simulink model "ToLinearize"  (R2018a)
settings: Solver=VariableStepAuto  StartTime=0.0  StopTime=100  RelTol=1e-3
values from neighbouring files (symbols this model uses):
  B_p = 0.01325    [heli_parameters.m]
  B_y = 0.8513    [heli_parameters.m]
  F_cpp = 1    [heli_parameters.m]
  F_cpy = 1    [heli_parameters.m]
  F_cyp = 1    [heli_parameters.m]
  F_cyy = 1    [heli_parameters.m]
  g = 9.81    [Spoustec_simu.m]    (also in heli_parameters.m)
  h = 0.00714    [Spoustec_simu.m]    (also in heli_parameters.m)
  J_eqp = 0.0332    [heli_parameters.m]
  J_eqy = 0.0371    [heli_parameters.m]
  K_pp = 0.02638    [heli_parameters.m]
  K_py = 0.00189    [heli_parameters.m]
  K_yp = 0.002096    [heli_parameters.m]
  K_yy = 0.01871    [heli_parameters.m]
  l_mc = 0.0122    [heli_parameters.m]
  m = 1.3872    [Spoustec_simu.m]    (also in heli_parameters.m)
libraries: mpclib x2, cstblocks x1
settings Model: Creator=ja  LastModifiedBy=ja

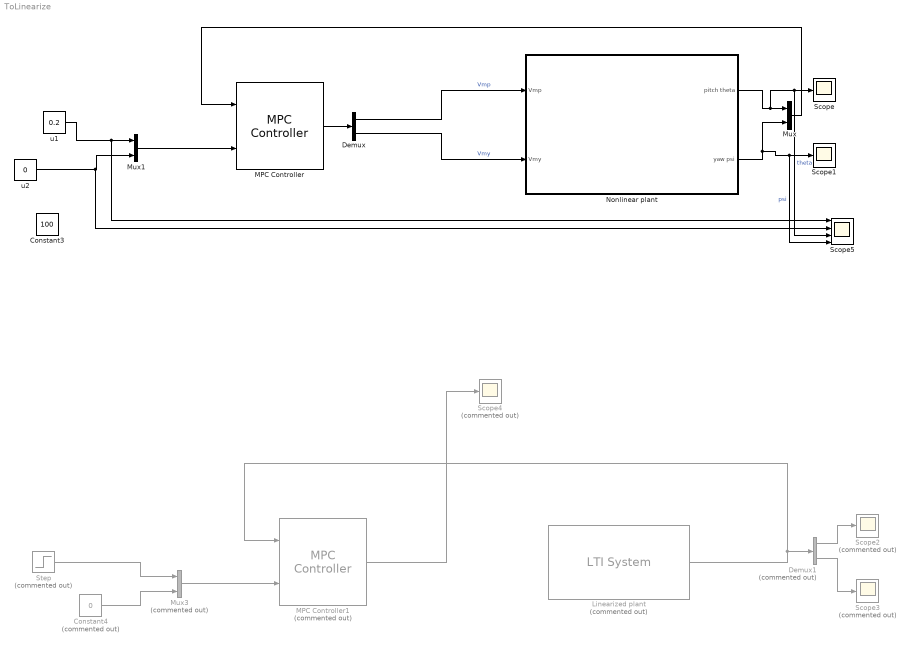
== system ToLinearize ==
  Constant3 : Constant  Value=100
  Constant4 : Constant  Commented=on  Value=0
  Demux : Demux  Outputs=2
  Demux1 : Demux  Commented=on  Outputs=2
  Linearized plant : cstblocks/LTI System  Commented=on  sys=plant  IC=[]
  MPC Controller : mpclib/MPC Controller  SCDEnableBlockLinearizationSpecification=on  mpcobj=mpc1  is_multiple=0  enable_value=0  return_u0=off  updateMPCinCallerWorkspace=on  ref_from_ws=off  ref_signal_name=[]  ref_preview=off  md_from_ws=off  md_signal_name=[]  md_preview=off  from_project=off  project_file=MPCtask.mat  md_inport=off  mv_inport=off  cost_outport=off  return_sequence=off  return_qpstatus=off  return_state=off  state_inport=off  lims_inport=off  cc_inport=off  ywt_inport=off  is_designfromscratch=0  uwt_inport=off  duwt_inport=off  rhoeps_inport=off  uref_inport=off  n_ts=1  n_p=20  n_mv=2  n_md=0  n_ud=0  n_mo=2  n_uo=0  BlockDataType=double  SampleTimeInherited=off  switch_inport=off
  MPC Controller1 : mpclib/MPC Controller  Commented=on  SCDEnableBlockLinearizationSpecification=on  is_multiple=0  enable_value=0  return_u0=off  updateMPCinCallerWorkspace=on  ref_from_ws=off  ref_signal_name=[]  ref_preview=off  md_from_ws=off  md_signal_name=[]  md_preview=off  from_project=off  project_file=MPCtask.mat  md_inport=off  mv_inport=off  cost_outport=off  return_sequence=off  return_qpstatus=off  return_state=off  state_inport=off  lims_inport=off  cc_inport=off  ywt_inport=off  is_designfromscratch=0  uwt_inport=off  duwt_inport=off  rhoeps_inport=off  uref_inport=off  n_ts=1  n_p=20  n_mv=2  n_md=0  n_ud=0  n_mo=2  n_uo=0  BlockDataType=double  SampleTimeInherited=off  switch_inport=off
  Mux : Mux  Inputs=2
  Mux1 : Mux  Inputs=2
  Mux3 : Mux  Commented=on  Inputs=2
  Nonlinear plant : Subsystem
      mask Display: image('Dynamics-of-2DOF-Helicopter.png');
  Scope : Scope
  Scope1 : Scope
  Scope2 : Scope  Commented=on
  Scope3 : Scope  Commented=on
  Scope4 : Scope  Commented=on
  Scope5 : Scope  NumInputPorts=4
  Step : Step  Commented=on  After=0.5  SampleTime=0
  u1 : Constant  Value=0.2
  u2 : Constant  Value=0
  wires:
  Demux/1 -> Nonlinear plant/1("Vmp ")  "Vmp"
  Demux/2 -> Nonlinear plant/2("Vmy ")  "Vmy"
  Nonlinear plant/1(pitch theta) -> Scope5/3, Scope/1, Mux/1  "theta"
  Nonlinear plant/2("yaw psi ") -> Scope5/4, Scope1/1, Mux/2  "psi"
  Mux/1 -> MPC Controller/1
  Mux1/1 -> MPC Controller/2
  u2/1 -> Scope5/2, Mux1/2
  Mux3/1 -> MPC Controller1/2
  Linearized plant/1 -> Demux1/1, MPC Controller1/1
  Step/1 -> Mux3/1
  Constant4/1 -> Mux3/2
  Demux1/1 -> Scope2/1
  Demux1/2 -> Scope3/1
  MPC Controller1/1 -> Scope4/1
  MPC Controller/1 -> Demux/1
  u1/1 -> Scope5/1, Mux1/1

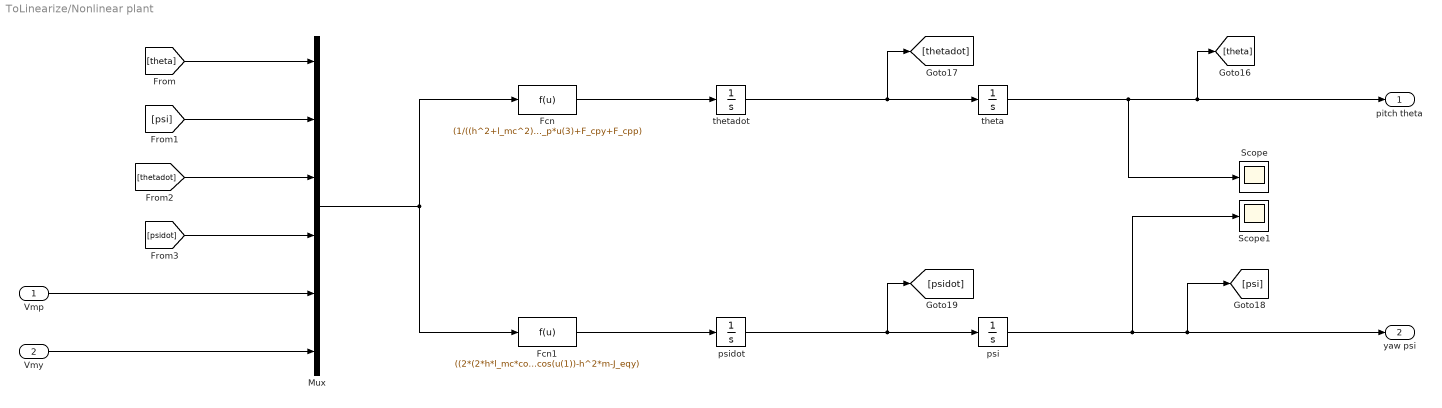
== system ToLinearize/Nonlinear plant ==
  "Vmp " : Inport
  "Vmy " : Inport  Port=2
  Fcn : Fcn  Expr=(1/((h^2+l_mc^2)*m+J_eqp))*(2*m*(h*l_mc*cos(u(1))^2+sin(u(1))*(h^2/2-l_mc^2/2)*cos(u(1))-(h*l_mc)/2)*u(4)^2-cos(u(1))*g*l_mc*m-sin(u(1))*g*h*m+K_pp*u(5)+K_py*u(6)-B_p*u(3)+F_cpy+F_cpp)
  Fcn1 : Fcn  Expr=((2*(2*h*l_mc*cos(u(1))^2+sin(u(1))*(h^2-l_mc^2)*cos(u(1))-h*l_mc)*m*u(3)+B_y)*u(4)-cos(u(1))*(K_yy*u(6)+K_yp*u(5)+F_cyp+F_cyy))/(m*(h^2-l_mc^2)*cos(u(1))^2-2*sin(u(1))*h*m*l_mc*cos(u(1))-h^2*m-J_eqy)
  Mux : Mux  Inputs=6
  Scope : Scope
  Scope1 : Scope
  psi : Integrator
  psidot : Integrator
  theta : Integrator
  thetadot : Integrator
  pitch theta : Outport
  "yaw psi " : Outport  Port=2
  wires:
  [psi] -> Mux/2
  Fcn/1 -> thetadot/1
  "Vmp "/1 -> Mux/5
  Mux/1 -> Fcn1/1, Fcn/1
  [thetadot] -> Mux/3
  psidot/1 -> [psidot], psi/1
  psi/1 -> Scope1/1, "yaw psi "/1, [psi]
  Fcn1/1 -> psidot/1
  "Vmy "/1 -> Mux/6
  [theta] -> Mux/1
  thetadot/1 -> [thetadot], theta/1
  theta/1 -> Scope/1, pitch theta/1, [theta]
  [psidot] -> Mux/4
